simulink model "write_point_cloud"  (R2018a)
settings: Solver=FixedStepAuto  StartTime=0.0  StopTime=Inf  RelTol=1e-3
model workspace (MAT data in the model file):
  SL_ROS_VariableLengthArrays_MaxSizes.CommonInfo.ArrayTruncateAction = 'EmitWarning'
  SL_ROS_VariableLengthArrays_MaxSizes.MsgTypeMap = containers.Map
  SL_ROS_VariableLengthArrays_MaxSizes.MsgTypeMap.serialization.keys = {'sensor_msgs/Image', 'sensor_msgs/PointCloud2'}
  SL_ROS_VariableLengthArrays_MaxSizes.MsgTypeMap.serialization.values{1}(1).PropertyName = 'Data'
  SL_ROS_VariableLengthArrays_MaxSizes.MsgTypeMap.serialization.values{1}(1).DataType = 'uint8'
  SL_ROS_VariableLengthArrays_MaxSizes.MsgTypeMap.serialization.values{1}(1).MaxLength = 921600
  SL_ROS_VariableLengthArrays_MaxSizes.MsgTypeMap.serialization.values{1}(2).PropertyName = 'Encoding'
  SL_ROS_VariableLengthArrays_MaxSizes.MsgTypeMap.serialization.values{1}(2).DataType = 'uint8'
  SL_ROS_VariableLengthArrays_MaxSizes.MsgTypeMap.serialization.values{1}(2).MaxLength = 128
  SL_ROS_VariableLengthArrays_MaxSizes.MsgTypeMap.serialization.values{2}(1).PropertyName = 'Data'
  SL_ROS_VariableLengthArrays_MaxSizes.MsgTypeMap.serialization.values{2}(1).DataType = 'uint8'
  SL_ROS_VariableLengthArrays_MaxSizes.MsgTypeMap.serialization.values{2}(1).MaxLength = 9830400
  SL_ROS_VariableLengthArrays_MaxSizes.MsgTypeMap.serialization.values{2}(2).PropertyName = 'Fields'
  SL_ROS_VariableLengthArrays_MaxSizes.MsgTypeMap.serialization.values{2}(2).DataType = 'sensor_msgs/PointField'
  SL_ROS_VariableLengthArrays_MaxSizes.MsgTypeMap.serialization.values{2}(2).MaxLength = 16
  SL_ROS_VariableLengthArrays_MaxSizes.MsgTypeMap.serialization.uniformity = 0
  SL_ROS_VariableLengthArrays_MaxSizes.MsgTypeMap.serialization.keyType = 'char'
  SL_ROS_VariableLengthArrays_MaxSizes.MsgTypeMap.serialization.valueType = 'any'
libraries: robotlib x2, simulink x1
settings Model: Creator=The MathWorks, Inc.  LastModifiedBy=tkikawad
settings OptimizationCC: EnhancedBackFolding=on  PassReuseOutputArgsAs=Individual arguments  MaxStackSize=64  OptimizeBlockOrder=speed  DifferentSizesBufferReuse=on  OptimizationCustomize=off
settings DebuggingCC: ParameterTunabilityLossMsg=error
settings HardwareCC: ProdBitPerLong=64  ProdHWDeviceType=Intel->x86-64 (Linux 64)
settings SFSimCC: MATLABDynamicMemAlloc=off
settings RTWCC: SystemTargetFile=ert.tlc  HardwareBoard=Robot Operating System (ROS)  TLCOptions="-aInlineSetEventsForThisBaseRateFcn=TLC_FALSE -aSuppressMultiTaskScheduler=TLC_FALSE  -aRateBasedStepFcn=0"  TemplateMakefile=ert_default_tmf  GenerateReport=on  Toolchain=Catkin  IncludeHyperlinkInReport=on  LaunchReport=on  TargetLang=C++  GenerateTraceInfo=on  GenerateTraceReport=on  GenerateTraceReportSl=on  GenerateTraceReportSf=on  GenerateTraceReportEml=on
settings CodeAppCC: ForceParamTrailComments=on  IgnoreCustomStorageClasses=off  OperatorAnnotations=on  SimulinkDataObjDesc=on  SFDataObjDesc=on  InsertBlockDesc=on

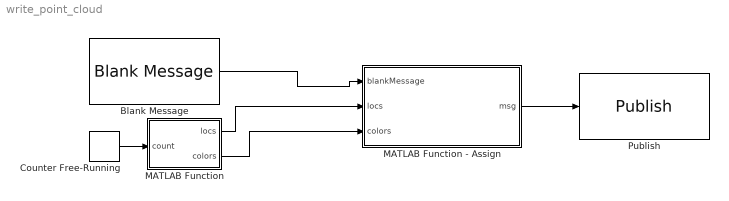
== system write_point_cloud ==
  Blank Message : robotlib/Blank Message  SourceLibraryInfo=This block requires Robotics System Toolbox  messageType=sensor_msgs/PointCloud2  SampleTime=inf
      settings: SourceProductBaseCode=RO
  Counter Free-Running : simulink/Sources/Counter Free-Running  NumBits=16  tsamp=-1
  MATLAB Function : MATLAB Function  TreatAsAtomicUnit=on
  MATLAB Function - Assign : MATLAB Function  TreatAsAtomicUnit=on
  Publish : robotlib/Publish  SourceLibraryInfo=This block requires Robotics System Toolbox  topicSource=Specify your own  topic=/ptcloud_test  messageType=sensor_msgs/PointCloud2  messageQueueLength=1
      settings: SourceProductBaseCode=RO
  wires:
  Blank Message/1 -> MATLAB Function - Assign/1(blankMessage)
  MATLAB Function - Assign/1(msg) -> Publish/1
  MATLAB Function/2(colors) -> MATLAB Function - Assign/3(colors)
  MATLAB Function/1(locs) -> MATLAB Function - Assign/2(locs)
  Counter Free-Running/1 -> MATLAB Function/1(count)

== matlab function write_point_cloud/MATLAB Function ==
  data: count input; locs output; colors output
function [locs,colors] = fcn(count)
count = double(count);
center = [160 120]/2;
[X,Y] = meshgrid(1:160,1:120);
Z = 10*sin((X-count-center(1))/10) + 10*cos((Y--center(2))/20) + 20;
locs = cat(3,X,Y,Z);
colors = im2uint8(hsv2rgb(cat(3,Z/40,ones(size(Z,1),size(Z,2),2))));

== matlab function write_point_cloud/MATLAB Function - Assign ==
  data: blankMessage input SL_Bus_write_point_cloud_sensor_msgs_PointCloud2; locs input; msg output SL_Bus_write_point_cloud_sensor_msgs_PointCloud2; colors input
function msg = assignNestedArrayMessages(blankMessage,locs,colors)
%#codegen

% To set datatype of MSG output:
%  1. Create buses for this model: robotics.ros.createSimulinkBus(gcs)
%  1. Click "Edit Data" in  Toolstrip to open "Ports and Data Manager"
%  2. Select MSG and set datatype to "Bus: SL_Bus_<modelname>_<messageType>"
% See: 
% http://www.mathworks.com/help/simulink/ug/create-structures-in-matlab-function-blocks.html

blankMessage.Height = uint32(size(locs,1));
blankMessage.Width = uint32(size(locs,2));
blankMessage.PointStep = uint32(32);
blankMessage.RowStep = blankMessage.Width * blankMessage.PointStep;
blankMessage.Fields_SL_Info.CurrentLength = uint32(4);
blankMessage.Fields(1).Name(1) = uint8('x');
blankMessage.Fields(1).Name_SL_Info.CurrentLength = uint32(1);
blankMessage.Fields(1).Offset = uint32(0);
blankMessage.Fields(1).Datatype = uint8(7);
blankMessage.Fields(1).Count = uint32(1);
blankMessage.Fields(2).Name(1) = uint8('y');
blankMessage.Fields(2).Name_SL_Info.CurrentLength = uint32(1);
blankMessage.Fields(2).Offset = uint32(4);
blankMessage.Fields(2).Datatype = uint8(7);
blankMessage.Fields(2).Count = uint32(1);
blankMessage.Fields(3).Name(1) = uint8('z');
blankMessage.Fields(3).Name_SL_Info.CurrentLength = uint32(1);
blankMessage.Fields(3).Offset = uint32(8);
blankMessage.Fields(3).Datatype = uint8(7);
blankMessage.Fields(3).Count = uint32(1);
blankMessage.Fields(4).Name(1:3) = uint8('rgb');
blankMessage.Fields(4).Name_SL_Info.CurrentLength = uint32(3);
blankMessage.Fields(4).Offset = uint32(16);
blankMessage.Fields(4).Datatype = uint8(7);
blankMessage.Fields(4).Count = uint32(1);

locs = reshape(permute(locs,[2 1 3]),[],3);
colors = uint32(reshape(permute(colors,[2 1 3]),[],3));
rgb = typecast(colors(:,1)*2^16+colors(:,2)*2^8+colors(:,3),'single');
data = [locs zeros(size(locs,1),1,'single') rgb zeros(size(locs,1),3,'single')];
dataPacked = reshape(permute(data,[2 1]),[],1);
dataCasted = typecast(dataPacked,'uint8');
blankMessage.Data(1:numel(dataCasted)) = dataCasted;
blankMessage.Data_SL_Info.CurrentLength = uint32(numel(dataCasted));

msg = blankMessage;
